simulink model "DIPC4M"  (R2015a)
settings: Solver=ode3  SolverMode=SingleTasking  StartTime=0.0  StopTime=3  FixedStep=1e-3  RelTol=1e-7
values from neighbouring files (symbols this model uses):
  alpha = 1.5    [CaViInit.m]    (also in CaccavaleVillani.m = 2)
  d1 = 1000    [CaViInit.m]    (also in CaccavaleVillani.m = 100)
  delta1 = 80    [CaViInit.m]    (also in CaccavaleVillani.m = 100)
  deltao = 10    [CaViInit.m]    (also in CaccavaleVillani.m = 2000)
  Do = 1500    [CaViInit.m]    (also in CaccavaleVillani.m = 2000)
  g = [0;0;-9.81]    [CaViInit.m]    (also in CaccavaleVillani.m)
  j0 = 0.2    [CaViInit.m]    (also in CaccavaleVillani.m = 1)
  j1 = 2    [CaViInit.m]    (also in CaccavaleVillani.m = 1)
  j1d = 1.00*j1    (= 2)    [CaViInit.m]    (also in CaccavaleVillani.m = 1)
  j2 = 2    [CaViInit.m]    (also in CaccavaleVillani.m = 1)
  j2d = 1.00*j2    (= 2)    [CaViInit.m]    (also in CaccavaleVillani.m = 1)
  j3 = 2    [CaViInit.m]    (also in CaccavaleVillani.m = 1)
  j3d = 1.00*j3    (= 2)    [CaViInit.m]    (also in CaccavaleVillani.m = 1)
  j4 = 2    [CaViInit.m]    (also in CaccavaleVillani.m = 1)
  j4d = 1.00*j4    (= 2)    [CaViInit.m]    (also in CaccavaleVillani.m = 1)
  k1 = 400    [CaViInit.m]    (also in CaccavaleVillani.m = 10000)
  K_o = 700    [CaViInit.m]    (also in CaccavaleVillani.m = 10000)
  kappa1 = 2    [CaViInit.m]    (also in CaccavaleVillani.m = 250)
  kappa_o = 5    [CaViInit.m]    (also in CaccavaleVillani.m = 10000)
  kpr = 150    [CaViInit.m]    (also in CaccavaleVillani.m = 10000)
  kpt = 50    [CaViInit.m]    (also in CaccavaleVillani.m = 50000)
  kv = 300    [CaccavaleVillani.m]
  m0 = 1.4    [CaViInit.m]    (also in CaccavaleVillani.m = 10)
  m1 = 2    [CaViInit.m]    (also in CaccavaleVillani.m = 10)
  m1d = 1.00*m1    (= 2)    [CaViInit.m]    (also in CaccavaleVillani.m = 10)
  m2 = 2    [CaViInit.m]    (also in CaccavaleVillani.m = 10)
  m2d = 1.00*m2    (= 2)    [CaViInit.m]    (also in CaccavaleVillani.m = 10)
  m3 = 2    [CaViInit.m]    (also in CaccavaleVillani.m = 10)
  m3d = 1.00*m3    (= 2)    [CaViInit.m]    (also in CaccavaleVillani.m = 10)
  m4 = 2    [CaViInit.m]    (also in CaccavaleVillani.m = 10)
  m4d = 1.00*m4    (= 2)    [CaViInit.m]    (also in CaccavaleVillani.m = 10)
  r = 0.4*[1; 0; 0 ... (first row only)    [CaViInit.m]    (also in CaccavaleVillani.m = [1; 0; 0)
libraries: aerolibutil x24, dspinverses x3, aerolibtransform2 x2, simulink x2
(part 1 of 2)
settings Model: CovSFcnEnable=off  Creator=Martin  LastModifiedBy=mangerer
settings SolverCC: ZeroCrossAlgorithm=Adaptive  AlgebraicLoopSolver=LineSearch
settings DataIOCC: LimitDataPoints=off
settings OptimizationCC: BlockReduction=off  BooleanDataType=off
settings DebuggingCC: SaveWithParameterizedLinksMsg=none  UnderspecifiedInitializationDetection=Classic  MergeDetectMultiDrivingBlocksExec=none  SignalResolutionControl=TryResolveAllWithWarning
settings HardwareCC: TargetUnknown=on

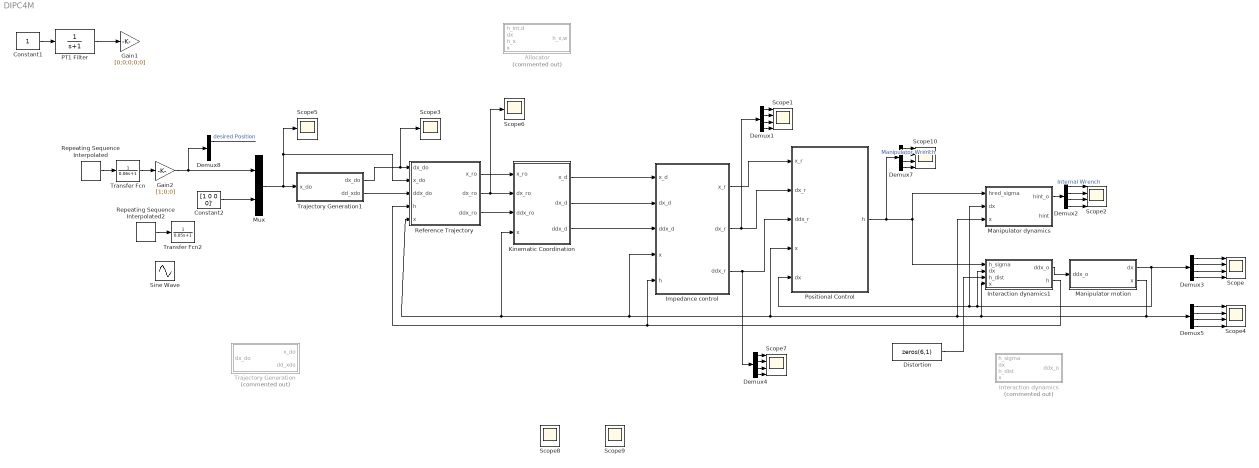
== system DIPC4M ==
  Allocator : Subsystem  Commented=on
  Constant1 : Constant
  Constant2 : Constant  Value=[1 0 0 0]'
  Demux{1..5,7} (6 alike) : Demux
  Demux8 : Demux  Outputs=3
  Distortion : Constant  Value=zeros(6,1)
  Gain1 : Gain  Gain=[0;0;0;0;0]
  Gain2 : Gain  Gain=[1;0;0]
  Impedance control : Subsystem
  Interaction dynamics : Subsystem  Commented=on
  Interaction dynamics1 : Subsystem
  Kinematic Coordination : Subsystem
  Manipulator dynamics : Subsystem
  Manipulator motion : Subsystem
  Mux : Mux  Inputs=2
  PT1 Filter : TransferFcn  Denominator=[1 1]
  Positional Control : Subsystem
  Reference Trajectory : Subsystem
  Repeating Sequence Interpolated : simulink/Sources/Repeating Sequence Interpolated  OutValues=[0 0 2 2 4 4 -2 -2 0 0].'  TimeValues=[0 0.1 0.14 0.9 0.96 1.8 1.95 2.4 2.6 3].'  LookUpMeth=Interpolation-Use End Values  tsamp=0.001  OutMin=[]  OutMax=[]  OutDataTypeStr=double  OutputDataTypeScalingMode=double  OutDataType=fixdt(0,8)  OutScaling=2^-10
  Repeating Sequence Interpolated2 : simulink/Sources/Repeating Sequence Interpolated  OutValues=[0 0 1 1 0 0].'  TimeValues=[0 0.1 1.5 2 2.5 3].'  LookUpMeth=Interpolation-Use End Values  tsamp=0.001  OutMin=[]  OutMax=[]  OutDataTypeStr=double  OutputDataTypeScalingMode=double  OutDataType=fixdt(0,8)  OutScaling=2^-10
  Scope{,1..2,4,7..10} (8 alike) : Scope  NumInputPorts=4
      Scope settings: ShowLegends=on  YMin=-1.5~-1.5~-1.5~-1.5  YMax=1.25~1.5~1.5~1.25
      Scope1 settings: ShowLegends=on  YMin=-2.5~-2.5~-3~-3  YMax=3~3~2.5~2.5
      Scope10 settings: ShowLegends=on  YMin=-30~-40~-40~-30  YMax=40~30~30~40  SaveName=ScopeData18
      Scope2 settings: ShowLegends=on  YMin=-1e-12~-1.5e-12~-7e-12~-3e-12  YMax=8e-12~3.5e-12~4e-12~4e-12  SaveName=ScopeData2
      Scope4 settings: ShowLegends=on  YMin=-1~-1~-0.5~-2  YMax=6~5~3.5~5  SaveName=ScopeData10
      Scope7 settings: ShowLegends=on  YMin=-3.5~-3.5~-3.5~-3.25  YMax=2~3~3~0.25  SaveName=ScopeData26
      Scope8 settings: Floating=on  ShowLegends=on  TimeRange=3  YMin=-3~-40~-10000~-0.005  YMax=5~30~10000~0.005  SaveName=ScopeData40
      Scope9 settings: Floating=on  ShowLegends=on  TimeRange=3  YMin=-0.2~-0.2~-30~-0.2  YMax=1.6~1.2~30~0.2  SaveName=ScopeData39
  Scope3 : Scope
      settings: SaveName=ScopeData8
  Scope5 : Scope
      settings: SaveName=ScopeData11
  Scope6 : Scope
      settings: YMin=-1  YMax=1  SaveName=ScopeData12
  Sine Wave : Sin  Frequency=1*pi  SampleTime=0
  Trajectory Generation : Subsystem  Commented=on
  Trajectory Generation1 : Subsystem
  Transfer Fcn : TransferFcn  Denominator=[0.06 1]
  Transfer Fcn2 : TransferFcn  Denominator=[0.05 1]
  wires:
  Manipulator dynamics/1(hint_o) -> Demux2/1
  Demux2/1 -> Scope2/1  "Internal Wrench"
  Demux2/2 -> Scope2/2
  Demux2/4 -> Scope2/4
  Demux3/1 -> Scope/1
  Demux3/2 -> Scope/2
  Demux3/3 -> Scope/3
  Demux3/4 -> Scope/4
  Demux5/1 -> Scope4/1
  Demux5/2 -> Scope4/2
  Demux5/3 -> Scope4/3
  Demux5/4 -> Scope4/4
  Demux7/1 -> Scope10/1  "Manipulator Wrench"
  Demux7/2 -> Scope10/2
  Demux7/3 -> Scope10/3
  Demux7/4 -> Scope10/4
  PT1 Filter/1 -> Gain1/1
  Manipulator motion/1(dx) -> Demux3/1, Positional Control/5(dx), Manipulator dynamics/2(dx), Interaction dynamics1/2(dx)
  Kinematic Coordination/1(x_d) -> Impedance control/1(x_d)
  Kinematic Coordination/3(ddx_d) -> Impedance control/3(ddx_d)
  Manipulator motion/2(x) -> Demux5/1, Interaction dynamics1/4(x), Manipulator dynamics/3(x), Positional Control/4(x), Kinematic Coordination/4(x), Reference Trajectory/5(x), Impedance control/4(x)
  Constant1/1 -> PT1 Filter/1
  Demux1/1 -> Scope1/1
  Demux1/2 -> Scope1/2
  Demux1/3 -> Scope1/3
  Demux1/4 -> Scope1/4
  Kinematic Coordination/2(dx_d) -> Impedance control/2(dx_d)
  Demux2/3 -> Scope2/3
  Interaction dynamics1/1(ddx_o) -> Manipulator motion/1(ddx_o)
  Distortion/1 -> Interaction dynamics1/3(h_dist)
  Reference Trajectory/1(x_ro) -> Kinematic Coordination/1(x_ro)
  Reference Trajectory/2(dx_ro) -> Scope6/1, Kinematic Coordination/2(dx_ro)
  Reference Trajectory/3(ddx_ro) -> Kinematic Coordination/3(ddx_ro)
  Impedance control/1(x_r) -> Positional Control/1(x_r)
  Impedance control/2(dx_r) -> Demux1/1, Positional Control/2(dx_r)
  Impedance control/3(ddx_r) -> Demux4/1, Positional Control/3(ddx_r)
  Positional Control/1(h) -> Demux7/1, Interaction dynamics1/1(h_sigma), Manipulator dynamics/1(hred_sigma)
  Demux4/1 -> Scope7/1
  Demux4/2 -> Scope7/2
  Demux4/3 -> Scope7/3
  Demux4/4 -> Scope7/4
  Repeating Sequence Interpolated2/1 -> Transfer Fcn2/1
  Mux/1 -> Scope5/1, Reference Trajectory/2(x_do), Trajectory Generation1/1(x_do)
  Trajectory Generation1/1(dx_do) -> Scope3/1, Reference Trajectory/1(dx_do)
  Trajectory Generation1/2(dd_xdo) -> Reference Trajectory/3(ddx_do)
  Gain2/1 -> Mux/1, Demux8/1
  Repeating Sequence Interpolated/1 -> Transfer Fcn/1
  Transfer Fcn/1 -> Gain2/1
  Demux8/1 -> ?  "desired Position"
  Constant2/1 -> Mux/2
  Interaction dynamics1/2(h) -> Reference Trajectory/4(h), Impedance control/5(h)

== system DIPC4M/Allocator ==
  h_int,d : Inport
  dx : Inport  Port=2
  h_x : Inport  Port=3
  x : Inport  Port=4
  Add : Sum  Inputs=-+
  Add1 : Sum
  Divide : Product  Inputs=*/*  Multiplication=Matrix(*)
  Divide1 : Product  Inputs=*/*  Multiplication=Matrix(*)
  Divide2 : Product  Inputs=*/*  Multiplication=Matrix(*)
  Inertia : Constant  Value=blkdiag(m1d*eye(3), j1d*eye(3), m2d*eye(3), j2d*eye(3), m3d*eye(3), j3d*eye(3), m4d*eye(3), j4d*eye(3))
  MATLAB Function : MATLAB Function  TreatAsAtomicUnit=on
  MATLAB Function1 : MATLAB Function  TreatAsAtomicUnit=on
  Math Function : Math  Operator=transpose  SaturateOnIntegerOverflow=on
  h_x,w : Outport
  wires:
  dx/1 -> MATLAB Function1/1(dx)
  Divide/1 -> h_x,w/1
  Math Function/1 -> Divide1/3, Divide/1
  MATLAB Function/1(Ared) -> Math Function/1, Divide2/1, Divide1/1
  Divide1/1 -> Divide/2
  Inertia/1 -> Divide1/2, Divide2/2
  MATLAB Function1/1(bred) -> Add/2
  Add/1 -> Divide/3
  Divide2/1 -> Add/1
  Add1/1 -> Divide2/3
  h_int,d/1 -> Add1/1
  h_x/1 -> Add1/2
  x/1 -> MATLAB Function1/2(x), MATLAB Function/1(x)

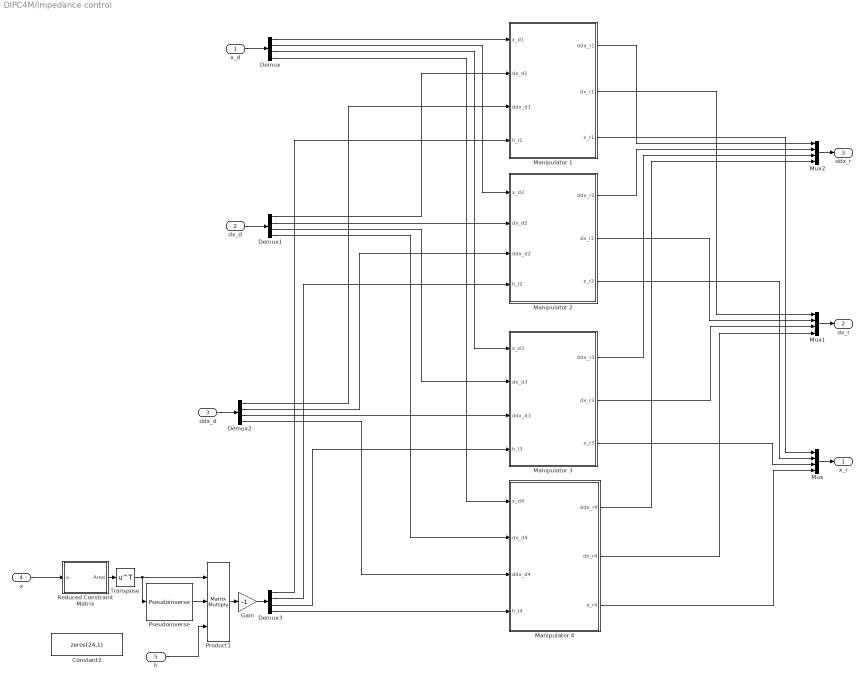
== system DIPC4M/Impedance control ==
  x_d : Inport
  dx_d : Inport  Port=2
  ddx_d : Inport  Port=3
  x : Inport  Port=4
  h : Inport  Port=5
  Constant2 : Constant  Value=zeros(24,1)
  Demux{,1..3} (4 alike) : Demux
  Gain : Gain  Gain=-1
  Manipulator 1 : Subsystem
  Manipulator 2 : Subsystem
  Manipulator 3 : Subsystem
  Manipulator 4 : Subsystem
  Mux : Mux
  Mux1 : Mux
  Mux2 : Mux
  Product1 : Product  Inputs=***  Multiplication=Matrix(*)
  Pseudoinverse : dspinverses/Pseudoinverse  wanterr=off
  Reduced Constraint Matrix : MATLAB Function  TreatAsAtomicUnit=on
  Transpose : Math  Operator=transpose  SaturateOnIntegerOverflow=on
  x_r : Outport
  dx_r : Outport  Port=2
  ddx_r : Outport  Port=3
  wires:
  ddx_d/1 -> Demux2/1
  dx_d/1 -> Demux1/1
  x_d/1 -> Demux/1
  Mux/1 -> x_r/1
  x/1 -> Reduced Constraint Matrix/1(x)
  Demux/1 -> Manipulator 1/1(x_d1)
  Demux/2 -> Manipulator 2/1(x_d2)
  Demux/3 -> Manipulator 3/1(x_d3)
  Demux1/1 -> Manipulator 1/2(dx_d1)
  Demux1/2 -> Manipulator 2/2(dx_d2)
  Demux1/3 -> Manipulator 3/2(dx_d3)
  Demux1/4 -> Manipulator 4/2(dx_d4)
  Demux/4 -> Manipulator 4/1(x_d4)
  Demux2/1 -> Manipulator 1/3(ddx_d1)
  Demux2/2 -> Manipulator 2/3(ddx_d2)
  Demux2/3 -> Manipulator 3/3(ddx_d3)
  Demux2/4 -> Manipulator 4/3(ddx_d4)
  Demux3/1 -> Manipulator 1/4(h_I1)
  Demux3/2 -> Manipulator 2/4(h_I2)
  Demux3/3 -> Manipulator 3/4(h_I3)
  Demux3/4 -> Manipulator 4/4(h_I4)
  Mux1/1 -> dx_r/1
  Mux2/1 -> ddx_r/1
  Manipulator 1/1(ddx_r1) -> Mux2/1
  Manipulator 2/1(ddx_r2) -> Mux2/2
  Manipulator 3/1(ddx_r3) -> Mux2/3
  Manipulator 4/1(ddx_r4) -> Mux2/4
  Manipulator 1/2(dx_r1) -> Mux1/1
  Manipulator 2/2(dx_r2) -> Mux1/2
  Manipulator 3/2(dx_r3) -> Mux1/3
  Manipulator 4/2(dx_r4) -> Mux1/4
  Manipulator 4/3(x_r4) -> Mux/4
  Manipulator 3/3(x_r3) -> Mux/3
  Manipulator 2/3(x_r2) -> Mux/2
  Manipulator 1/3(x_r1) -> Mux/1
  Pseudoinverse/1 -> Product1/2
  Reduced Constraint Matrix/1(Ared) -> Transpose/1
  Transpose/1 -> Product1/1, Pseudoinverse/1
  Product1/1 -> Gain/1
  Gain/1 -> Demux3/1
  h/1 -> Product1/3

== system DIPC4M/Interaction dynamics ==
  h_sigma : Inport
  dx : Inport  Port=2
  h_dist : Inport  Port=3
  x : Inport  Port=4
  Apparent Inertia : MATLAB Function  TreatAsAtomicUnit=on
  Centripetal Force : MATLAB Function  TreatAsAtomicUnit=on
  Coriolis Force : MATLAB Function  TreatAsAtomicUnit=on
  G h_sigma : Product  Multiplication=Matrix(*)
  GMb : Product  Inputs=***  Multiplication=Matrix(*)
  Grasp Matrix : MATLAB Function  TreatAsAtomicUnit=on
  Gravitation : Constant  Value=[-m0*g;zeros(3,1)]
  Inertia : Constant  Value=blkdiag(m1*eye(3), j1*eye(3), m2*eye(3), j2*eye(3), m3*eye(3), j3*eye(3), m4*eye(3), j4*eye(3))
  M_app^-1 h_o : Product  Inputs=/*  Multiplication=Matrix(*)
  "h_dist - h_g - j0 S(omega0) omega0 " : Sum  Inputs=+--
  h_o : Sum  Inputs=++-
  ddx_o : Outport
  wires:
  Grasp Matrix/1(G) -> G h_sigma/1, GMb/1, Apparent Inertia/1(G)
  Inertia/1 -> GMb/2, Apparent Inertia/2(M)
  Apparent Inertia/1(Mapp) -> M_app^-1 h_o/1
  h_o/1 -> M_app^-1 h_o/2
  G h_sigma/1 -> h_o/2
  h_sigma/1 -> G h_sigma/2
  "h_dist - h_g - j0 S(omega0) omega0 "/1 -> h_o/1
  h_dist/1 -> "h_dist - h_g - j0 S(omega0) omega0 "/1
  Gravitation/1 -> "h_dist - h_g - j0 S(omega0) omega0 "/2
  dx/1 -> Centripetal Force/1(dx), Coriolis Force/1(dx)
  Coriolis Force/1(hcoriolis) -> "h_dist - h_g - j0 S(omega0) omega0 "/3
  GMb/1 -> h_o/3
  Centripetal Force/1(b) -> GMb/3
  M_app^-1 h_o/1 -> ddx_o/1
  x/1 -> Centripetal Force/2(x), Grasp Matrix/1(x)

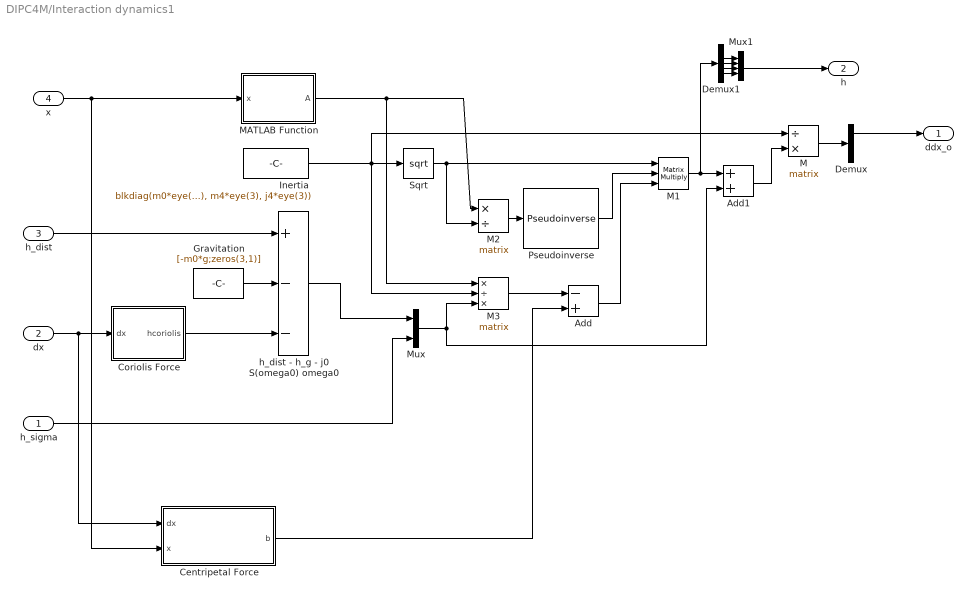
== system DIPC4M/Interaction dynamics1 ==
  h_sigma : Inport
  dx : Inport  Port=2
  h_dist : Inport  Port=3
  x : Inport  Port=4
  Add : Sum  Inputs=-+
  Add1 : Sum
  Centripetal Force : MATLAB Function  TreatAsAtomicUnit=on
  Coriolis Force : MATLAB Function  TreatAsAtomicUnit=on
  Demux : Demux  Outputs=5
  Demux1 : Demux  Outputs=5
  Gravitation : Constant  Value=[-m0*g;zeros(3,1)]
  Inertia : Constant  Value=blkdiag(m0*eye(3),j0*eye(3),m1*eye(3), j1*eye(3), m2*eye(3), j2*eye(3), m3*eye(3), j3*eye(3), m4*eye(3), j4*eye(3))
  M : Product  Inputs=/*  Multiplication=Matrix(*)
  M1 : Product  Inputs=***  Multiplication=Matrix(*)
  M2 : Product  Inputs=*/  Multiplication=Matrix(*)
  M3 : Product  Inputs=*/*  Multiplication=Matrix(*)
  MATLAB Function : MATLAB Function  TreatAsAtomicUnit=on
  Mux : Mux  Inputs=2
  Mux1 : Mux
  Pseudoinverse : dspinverses/Pseudoinverse  wanterr=off
  Sqrt : Sqrt  SaturateOnIntegerOverflow=on
  "h_dist - h_g - j0 S(omega0) omega0 " : Sum  Inputs=+--
  ddx_o : Outport
  h : Outport  Port=2
  wires:
  h_dist/1 -> "h_dist - h_g - j0 S(omega0) omega0 "/1
  Gravitation/1 -> "h_dist - h_g - j0 S(omega0) omega0 "/2
  dx/1 -> Centripetal Force/1(dx), Coriolis Force/1(dx)
  Coriolis Force/1(hcoriolis) -> "h_dist - h_g - j0 S(omega0) omega0 "/3
  x/1 -> MATLAB Function/1(x), Centripetal Force/2(x)
  Inertia/1 -> M/1, M3/2, Sqrt/1
  Sqrt/1 -> M2/2, M1/1
  MATLAB Function/1(A) -> M3/1, M2/1
  M2/1 -> Pseudoinverse/1
  Pseudoinverse/1 -> M1/2
  Add/1 -> M1/3
  Centripetal Force/1(b) -> Add/2
  M3/1 -> Add/1
  Mux/1 -> Add1/2, M3/3
  "h_dist - h_g - j0 S(omega0) omega0 "/1 -> Mux/1
  h_sigma/1 -> Mux/2
  M/1 -> Demux/1
  Demux/1 -> ddx_o/1
  M1/1 -> Demux1/1, Add1/1
  Add1/1 -> M/2
  Demux1/2 -> Mux1/1
  Demux1/3 -> Mux1/2
  Demux1/4 -> Mux1/3
  Demux1/5 -> Mux1/4
  Mux1/1 -> h/1

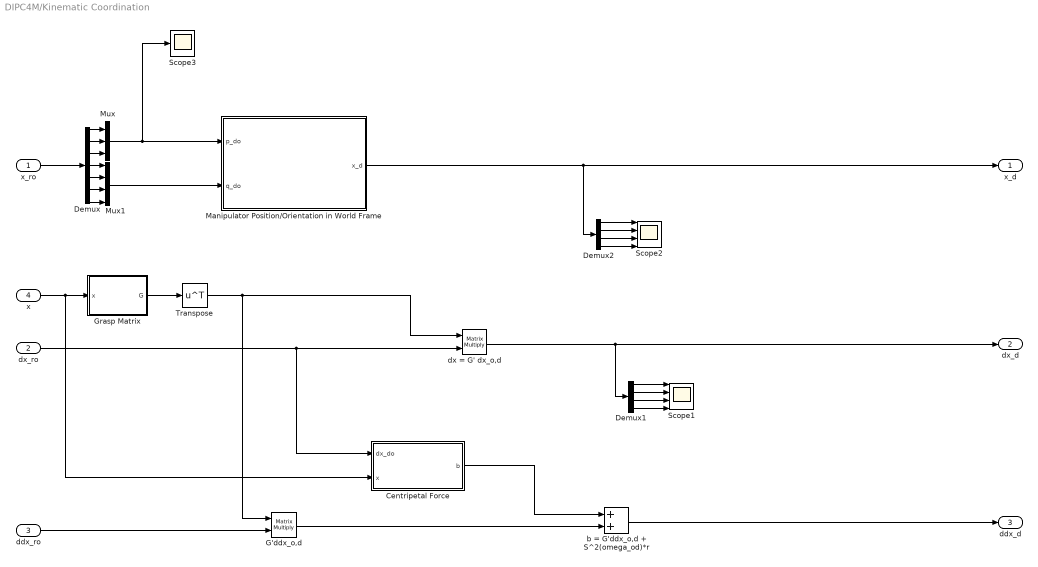
== system DIPC4M/Kinematic Coordination ==
  x_ro : Inport
  dx_ro : Inport  Port=2
  ddx_ro : Inport  Port=3
  x : Inport  Port=4
  Centripetal Force : MATLAB Function  TreatAsAtomicUnit=on
  Demux : Demux  Outputs=7
  Demux1 : Demux
  Demux2 : Demux
  G'ddx_o,d : Product  Multiplication=Matrix(*)
  Grasp Matrix : MATLAB Function  TreatAsAtomicUnit=on
  Manipulator Position/Orientation in World Frame : MATLAB Function  TreatAsAtomicUnit=on
  Mux : Mux  Inputs=3
  Mux1 : Mux
  Scope1 : Scope  NumInputPorts=4
      settings: ShowLegends=on  YMin=-1.5~-1.5~-1.5~-1.5  YMax=6~5.5~6~5.5  SaveName=ScopeData3
  Scope2 : Scope  NumInputPorts=4
      settings: ShowLegends=on  YMin=-1.5~-1.5~-1.5~-1.5  YMax=6~5.5~6~5.5  SaveName=ScopeData4
  Scope3 : Scope
      settings: ShowLegends=on  TimeRange=5  YMin=-0.25  YMax=0.175  SaveName=ScopeData30
  Transpose : Math  Operator=transpose  SaturateOnIntegerOverflow=on
  b = G'ddx_o,d + S^2(omega_od)*r : Sum
  dx = G' dx_o,d : Product  Multiplication=Matrix(*)
  x_d : Outport
  dx_d : Outport  Port=2
  ddx_d : Outport  Port=3
  wires:
  Grasp Matrix/1(G) -> Transpose/1
  Transpose/1 -> G'ddx_o,d/1, dx = G' dx_o,d/1
  dx = G' dx_o,d/1 -> Demux1/1, dx_d/1
  x_ro/1 -> Demux/1
  Demux/1 -> Mux/1
  Demux/2 -> Mux/2
  Demux/3 -> Mux/3
  Demux/5 -> Mux1/2
  Demux/6 -> Mux1/3
  Demux/7 -> Mux1/4
  Demux/4 -> Mux1/1
  Mux1/1 -> Manipulator Position/Orientation in World Frame/2(q_do)
  Mux/1 -> Scope3/1, Manipulator Position/Orientation in World Frame/1(p_do)
  Centripetal Force/1(b) -> b = G'ddx_o,d + S^2(omega_od)*r/1
  ddx_ro/1 -> G'ddx_o,d/2
  G'ddx_o,d/1 -> b = G'ddx_o,d + S^2(omega_od)*r/2
  b = G'ddx_o,d + S^2(omega_od)*r/1 -> ddx_d/1
  dx_ro/1 -> Centripetal Force/1(dx_do), dx = G' dx_o,d/2
  Demux1/1 -> Scope1/1
  Demux1/2 -> Scope1/2
  Demux1/3 -> Scope1/3
  Demux1/4 -> Scope1/4
  Manipulator Position/Orientation in World Frame/1(x_d) -> Demux2/1, x_d/1
  Demux2/1 -> Scope2/1
  Demux2/2 -> Scope2/2
  Demux2/3 -> Scope2/3
  Demux2/4 -> Scope2/4
  x/1 -> Centripetal Force/2(x), Grasp Matrix/1(x)

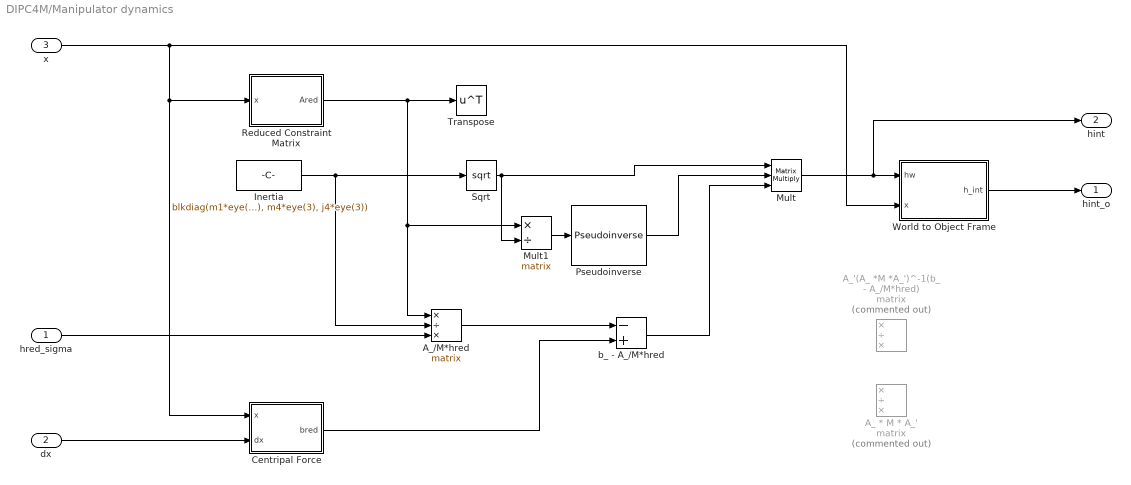
== system DIPC4M/Manipulator dynamics ==
  hred_sigma : Inport
  dx : Inport  Port=2
  x : Inport  Port=3
  A_ * M * A_' : Product  Commented=on  Inputs=*/*  Multiplication=Matrix(*)
  A_'(A_ *M *A_')^-1(b_ - A_/M*hred) : Product  Commented=on  Inputs=*/*  Multiplication=Matrix(*)
  A_/M*hred : Product  Inputs=*/*  Multiplication=Matrix(*)
  Centripal Force : MATLAB Function  TreatAsAtomicUnit=on
  Inertia : Constant  Value=blkdiag(m1*eye(3), j1*eye(3), m2*eye(3), j2*eye(3), m3*eye(3), j3*eye(3), m4*eye(3), j4*eye(3))
  Mult : Product  Inputs=***  Multiplication=Matrix(*)
  Mult1 : Product  Inputs=*/  Multiplication=Matrix(*)
  Pseudoinverse : dspinverses/Pseudoinverse  wanterr=off
  Reduced Constraint Matrix : MATLAB Function  TreatAsAtomicUnit=on
  Sqrt : Sqrt  SaturateOnIntegerOverflow=on
  Transpose : Math  Operator=transpose  SaturateOnIntegerOverflow=on
  World to Object Frame : MATLAB Function  TreatAsAtomicUnit=on
  b_ - A_/M*hred : Sum  Inputs=-+
  hint_o : Outport
  hint : Outport  Port=2
  wires:
  Reduced Constraint Matrix/1(Ared) -> Transpose/1, A_/M*hred/1, Mult1/1
  Inertia/1 -> Sqrt/1, A_/M*hred/2
  dx/1 -> Centripal Force/2(dx)
  A_/M*hred/1 -> b_ - A_/M*hred/1
  hred_sigma/1 -> A_/M*hred/3
  World to Object Frame/1(h_int) -> hint_o/1
  x/1 -> Centripal Force/1(x), Reduced Constraint Matrix/1(x), World to Object Frame/2(x)
  Centripal Force/1(bred) -> b_ - A_/M*hred/2
  Mult/1 -> hint/1, World to Object Frame/1(hw)
  b_ - A_/M*hred/1 -> Mult/3
  Sqrt/1 -> Mult1/2, Mult/1
  Mult1/1 -> Pseudoinverse/1
  Pseudoinverse/1 -> Mult/2

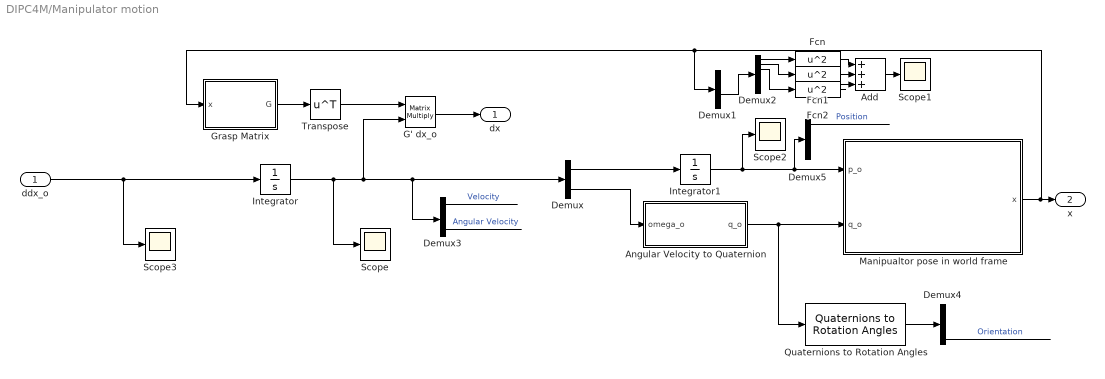
== system DIPC4M/Manipulator motion ==
  ddx_o : Inport
  Add : Sum  Inputs=+++
  Angular Velocity to Quaternion : Subsystem
  Demux : Demux  Outputs=2
  Demux1 : Demux
  Demux2 : Demux  Outputs=7
  Demux3 : Demux  Outputs=6
  Demux4 : Demux  Outputs=3
  Demux5 : Demux  Outputs=3
  Fcn : Fcn  Expr=u^2
  Fcn1 : Fcn  Expr=u^2
  Fcn2 : Fcn  Expr=u^2
  G' dx_o : Product  Multiplication=Matrix(*)
  Grasp Matrix : MATLAB Function  TreatAsAtomicUnit=on
  Integrator : Integrator  InitialCondition=zeros(6,1)
  Integrator1 : Integrator  InitialCondition=[0 0 0]'
  Manipualtor pose in world frame : MATLAB Function  TreatAsAtomicUnit=on
  Quaternions to Rotation Angles : aerolibtransform2/Quaternions to Rotation Angles  rotationOrder=XYZ
  Scope{,1..3} (4 alike) : Scope
      Scope settings: YMin=-1.1  YMax=1.1  SaveName=ScopeData14
      Scope1 settings: YMin=0  YMax=40  SaveName=ScopeData15
      Scope2 settings: YMin=-1  YMax=1  SaveName=ScopeData6
      Scope3 settings: SaveName=ScopeData7
  Transpose : Math  Operator=transpose  SaturateOnIntegerOverflow=on
  dx : Outport
  x : Outport  Port=2
  wires:
  ddx_o/1 -> Scope3/1, Integrator/1
  Integrator/1 -> Scope/1, G' dx_o/2, Demux3/1, Demux/1
  Grasp Matrix/1(G) -> Transpose/1
  Transpose/1 -> G' dx_o/1
  G' dx_o/1 -> dx/1
  Demux/2 -> Angular Velocity to Quaternion/1(omega_o)
  Demux/1 -> Integrator1/1
  Integrator1/1 -> Scope2/1, Demux5/1, Manipualtor pose in world frame/1(p_o)
  Manipualtor pose in world frame/1(x) -> Demux1/1, Grasp Matrix/1(x), x/1
  Angular Velocity to Quaternion/1(q_o) -> Quaternions to Rotation Angles/1, Manipualtor pose in world frame/2(q_o)
  Add/1 -> Scope1/1
  Fcn/1 -> Add/1
  Fcn1/1 -> Add/2
  Fcn2/1 -> Add/3
  Demux2/1 -> Fcn/1
  Demux2/2 -> Fcn1/1
  Demux2/3 -> Fcn2/1
  Demux1/3 -> Demux2/1
  Demux3/1 -> ?  "Velocity"
  Quaternions to Rotation Angles/1 -> Demux4/1
  Demux4/3 -> ?  "Orientation"
  Demux3/6 -> ?  "Angular Velocity"
  Demux5/1 -> ?  "Position"

== system DIPC4M/Positional Control ==
  x_r : Inport
  dx_r : Inport  Port=2
  ddx_r : Inport  Port=3
  x : Inport  Port=4
  dx : Inport  Port=5
  Add : Sum  Inputs=+++
  Add1 : Sum  Inputs=+-
  Manipulator Inertia : Constant  Value=blkdiag(m1*eye(3), j1*eye(3), m2*eye(3), j2*eye(3), m3*eye(3), j3*eye(3), m4*eye(3), j4*eye(3))
  Manipulator kv : Constant  Value=kv*eye(24)
  Product : Product  Multiplication=Matrix(*)
  Product1 : Product  Multiplication=Matrix(*)
  Subsystem : Subsystem
  h : Outport
  wires:
  Product/1 -> h/1
  Manipulator Inertia/1 -> Product/1
  Add/1 -> Product/2
  ddx_r/1 -> Add/3
  dx_r/1 -> Add1/1
  dx/1 -> Add1/2
  x/1 -> Subsystem/2(x)
  x_r/1 -> Subsystem/1(x_r)
  Subsystem/1(hk) -> Add/1
  Add1/1 -> Product1/2
  Manipulator kv/1 -> Product1/1
  Product1/1 -> Add/2

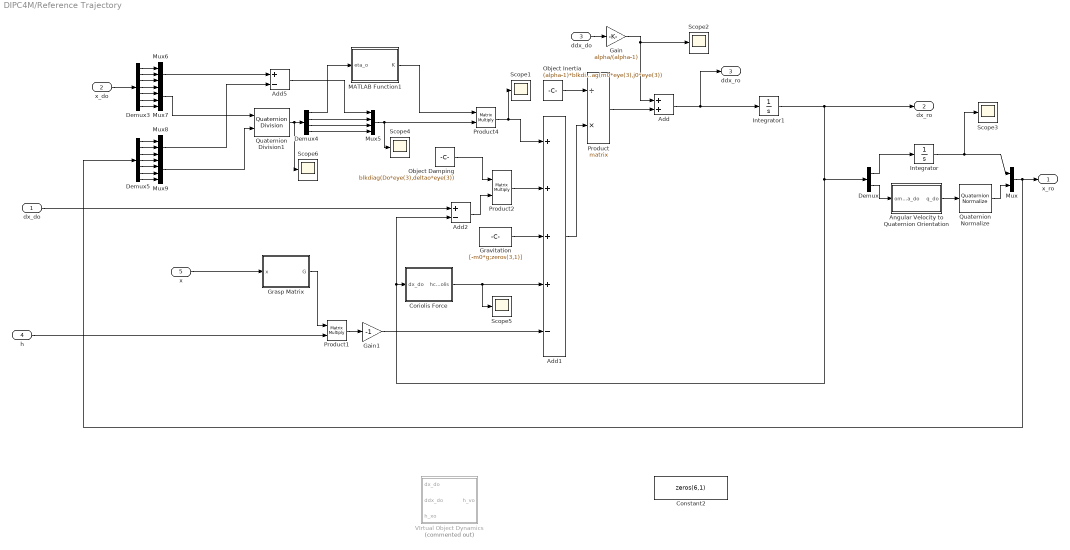
== system DIPC4M/Reference Trajectory ==
  dx_do : Inport
  x_do : Inport  Port=2
  ddx_do : Inport  Port=3
  h : Inport  Port=4
  x : Inport  Port=5
  Add : Sum
  Add1 : Sum  Inputs=++++-
  Add2 : Sum  Inputs=+-
  Add5 : Sum  Inputs=+-
  Angular Velocity to Quaternion Orientation : Subsystem
  Constant2 : Constant  Value=zeros(6,1)
  Coriolis Force : MATLAB Function  TreatAsAtomicUnit=on
  Demux : Demux  Outputs=2
  Demux3 : Demux  Outputs=7
  Demux4 : Demux
  Demux5 : Demux  Outputs=7
  Gain : Gain  Gain=alpha/(alpha-1)
  Gain1 : Gain  Gain=-1
  Grasp Matrix : MATLAB Function  TreatAsAtomicUnit=on
  Gravitation : Constant  Value=[-m0*g;zeros(3,1)]
  Integrator : Integrator  InitialCondition=zeros(3,1)
  Integrator1 : Integrator  InitialCondition=zeros(6,1)
  MATLAB Function1 : MATLAB Function  TreatAsAtomicUnit=on
  Mux : Mux  Inputs=2
  Mux5 : Mux
  Mux6 : Mux  Inputs=3
  Mux7 : Mux
  Mux8 : Mux  Inputs=3
  Mux9 : Mux
  Object Damping : Constant  Value=blkdiag(Do*eye(3),deltao*eye(3))
  Object Inertia : Constant  Value=(alpha-1)*blkdiag(m0*eye(3),j0*eye(3))
  Product : Product  Inputs=/*  Multiplication=Matrix(*)
  Product1 : Product  Multiplication=Matrix(*)
  Product2 : Product  Multiplication=Matrix(*)
  Product4 : Product  Multiplication=Matrix(*)
  Quaternion Division1 : aerolibutil/Quaternion Division
  Quaternion Normalize : aerolibutil/Quaternion Normalize
  Scope{1..6} (6 alike) : Scope
      Scope1 settings: YMin=-325  YMax=100  SaveName=ScopeData23
      Scope2 settings: SaveName=ScopeData25
      Scope3 settings: ShowLegends=on  TimeRange=5  YMin=-0.15  YMax=0.01  SaveName=ScopeData31
      Scope4 settings: YMin=-0.4  YMax=0.25  SaveName=ScopeData27
      Scope5 settings: ShowLegends=on  TimeRange=5  YMin=-15  YMax=12.5  SaveName=ScopeData32
      Scope6 settings: YMin=-0.05  YMax=1  SaveName=ScopeData28
  VIrtual Object Dynamics : Subsystem  Commented=on
  x_ro : Outport
  dx_ro : Outport  Port=2
  ddx_ro : Outport  Port=3
  wires:
  Object Inertia/1 -> Product/1
  Add/1 -> ddx_ro/1, Integrator1/1
  Add1/1 -> Product/2
  MATLAB Function1/1(K) -> Product4/1
  Demux4/1 -> MATLAB Function1/1(eta_o)
  Add5/1 -> Mux5/1
  Demux4/2 -> Mux5/2
  Demux4/3 -> Mux5/3
  Demux4/4 -> Mux5/4
  x_do/1 -> Demux3/1
  Demux3/2 -> Mux6/2
  Demux3/1 -> Mux6/1
  Demux3/3 -> Mux6/3
  Demux3/4 -> Mux7/1
  Demux3/5 -> Mux7/2
  Demux3/6 -> Mux7/3
  Demux3/7 -> Mux7/4
  Demux5/2 -> Mux8/2
  Demux5/1 -> Mux8/1
  Demux5/3 -> Mux8/3
  Demux5/4 -> Mux9/1
  Demux5/5 -> Mux9/2
  Demux5/6 -> Mux9/3
  Demux5/7 -> Mux9/4
  Quaternion Division1/1 -> Scope6/1, Demux4/1
  Mux5/1 -> Scope4/1, Product4/2
  Product4/1 -> Scope1/1, Add1/1
  Mux6/1 -> Add5/1
  Mux7/1 -> Quaternion Division1/1
  Mux8/1 -> Add5/2
  Demux/2 -> Angular Velocity to Quaternion Orientation/1(omega_do)
  Demux/1 -> Integrator/1
  Integrator/1 -> Scope3/1, Mux/1
  Mux/1 -> Demux5/1, x_ro/1
  Grasp Matrix/1(G) -> Product1/1
  ddx_do/1 -> Gain/1
  Gain/1 -> Scope2/1, Add/1
  Product/1 -> Add/2
  Product2/1 -> Add1/2
  Object Damping/1 -> Product2/1
  Add2/1 -> Product2/2
  dx_do/1 -> Add2/1
  Gravitation/1 -> Add1/3
  Coriolis Force/1(hcoriolis) -> Scope5/1, Add1/4
  Integrator1/1 -> Add2/2, Coriolis Force/1(dx_do), Demux/1, dx_ro/1
  x/1 -> Grasp Matrix/1(x)
  Angular Velocity to Quaternion Orientation/1(q_do) -> Quaternion Normalize/1
  Mux9/1 -> Quaternion Division1/2
  Quaternion Normalize/1 -> Mux/2
  Product1/1 -> Gain1/1
  Gain1/1 -> Add1/5
  h/1 -> Product1/2

== system DIPC4M/Trajectory Generation ==
  dx_do : Inport
  Angular Velocity to Quaternion Orientation : Subsystem
  Demux : Demux  Outputs=2
  Demux4 : Demux  Outputs=3
  Derivative : Derivative
  Integrator : Integrator  InitialCondition=zeros(3,1)
  Mux : Mux  Inputs=2
  Quaternion Normalize : aerolibutil/Quaternion Normalize
  Quaternions to Rotation Angles : aerolibtransform2/Quaternions to Rotation Angles  rotationOrder=XYZ
  Scope : Scope
      settings: SaveName=ScopeData16
  x_do : Outport
  dd_xdo : Outport  Port=2
  wires:
  dx_do/1 -> Derivative/1, Demux/1
  Demux/2 -> Angular Velocity to Quaternion Orientation/1(omega_do)
  Demux/1 -> Integrator/1
  Angular Velocity to Quaternion Orientation/1(q_do) -> Quaternion Normalize/1
  Integrator/1 -> Mux/1
  Mux/1 -> x_do/1
  Derivative/1 -> dd_xdo/1
  Quaternion Normalize/1 -> Quaternions to Rotation Angles/1, Scope/1, Mux/2
  Quaternions to Rotation Angles/1 -> Demux4/1
  Demux4/3 -> ?  "desired Orientation"

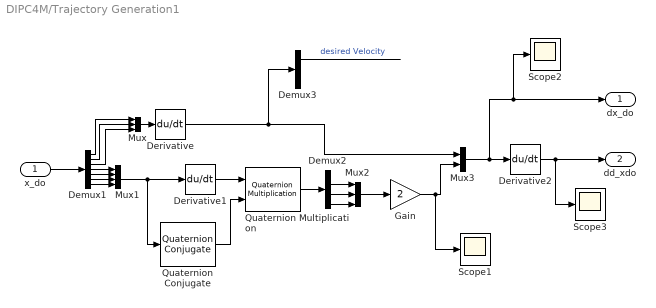
== system DIPC4M/Trajectory Generation1 ==
  x_do : Inport
  Demux1 : Demux  Outputs=7
  Demux2 : Demux
  Demux3 : Demux  Outputs=3
  Derivative : Derivative
  Derivative1 : Derivative
  Derivative2 : Derivative
  Gain : Gain  Gain=2
  Mux : Mux  Inputs=3
  Mux1 : Mux
  Mux2 : Mux  Inputs=3
  Mux3 : Mux  Inputs=2
  Quaternion Conjugate : aerolibutil/Quaternion Conjugate
  Quaternion Multiplication : aerolibutil/Quaternion Multiplication
  Scope1 : Scope
      settings: ShowLegends=on  YMin=0  YMax=2  SaveName=ScopeData10
  Scope2 : Scope
      settings: YMin=0  YMax=2  SaveName=ScopeData11
  Scope3 : Scope
      settings: YMin=-1.5e-09  YMax=1.5e-09  SaveName=ScopeData8
  dx_do : Outport
  dd_xdo : Outport  Port=2
  wires:
  x_do/1 -> Demux1/1
  Demux1/1 -> Mux/1
  Demux1/2 -> Mux/2
  Demux1/3 -> Mux/3
  Demux1/4 -> Mux1/1
  Demux1/5 -> Mux1/2
  Demux1/6 -> Mux1/3
  Demux1/7 -> Mux1/4
  Mux/1 -> Derivative/1
  Mux1/1 -> Quaternion Conjugate/1, Derivative1/1
  Derivative1/1 -> Quaternion Multiplication/1
  Quaternion Conjugate/1 -> Quaternion Multiplication/2
  Quaternion Multiplication/1 -> Demux2/1
  Demux2/4 -> Mux2/3
  Demux2/3 -> Mux2/2
  Demux2/2 -> Mux2/1
  Mux2/1 -> Gain/1
  Gain/1 -> Scope1/1, Mux3/2
  Derivative/1 -> Demux3/1, Mux3/1
  Mux3/1 -> Scope2/1, dx_do/1, Derivative2/1
  Derivative2/1 -> Scope3/1, dd_xdo/1
  Demux3/1 -> ?  "desired Velocity"

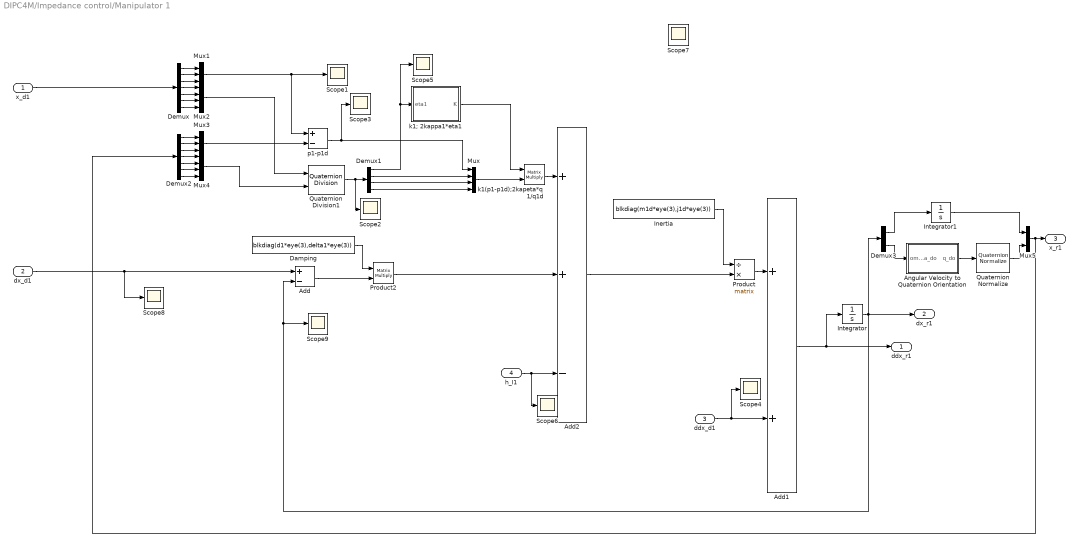
== system DIPC4M/Impedance control/Manipulator 1 ==
  x_d1 : Inport
  dx_d1 : Inport  Port=2
  ddx_d1 : Inport  Port=3
  h_I1 : Inport  Port=4
  Add : Sum  Inputs=+-
  Add1 : Sum
  Add2 : Sum  Inputs=++-
  Angular Velocity to Quaternion Orientation : Subsystem
  Damping : Constant  Value=blkdiag(d1*eye(3),delta1*eye(3))
  Demux : Demux  Outputs=7
  Demux1 : Demux
  Demux2 : Demux  Outputs=7
  Demux3 : Demux  Outputs=2
  Inertia : Constant  Value=blkdiag(m1d*eye(3),j1d*eye(3))
  Integrator : Integrator
  Integrator1 : Integrator  InitialCondition=r(1:3)
  Mux : Mux
  Mux1 : Mux  Inputs=3
  Mux2 : Mux
  Mux3 : Mux  Inputs=3
  Mux4 : Mux
  Mux5 : Mux  Inputs=2
  Product : Product  Inputs=/*  Multiplication=Matrix(*)
  Product2 : Product  Multiplication=Matrix(*)
  Quaternion Division1 : aerolibutil/Quaternion Division
  Quaternion Normalize : aerolibutil/Quaternion Normalize
  Scope{1..9} (9 alike) : Scope
      Scope1 settings: ShowLegends=on  TimeRange=5  YMin=2.77556e-17  YMax=1.05  SaveName=ScopeData29
      Scope2 settings: ShowLegends=on  TimeRange=5  YMin=-0.18  YMax=0.01  SaveName=ScopeData33
      Scope3 settings: ShowLegends=on  TimeRange=5  YMin=-0.18  YMax=0.01  SaveName=ScopeData21
      Scope4 settings: ShowLegends=on  TimeRange=5  YMin=-3.5  YMax=3  SaveName=ScopeData34
      Scope5 settings: ShowLegends=on  TimeRange=200  YMin=-50  YMax=125  SaveName=ScopeData24
      Scope6 settings: ShowLegends=on  TimeRange=5  YMin=-2.75e+09  YMax=1.5e+09  SaveName=ScopeData35
      Scope7 settings: ShowLegends=on  TimeRange=5  YMin=-0.18  YMax=0.01  SaveName=ScopeData36
      Scope8 settings: ShowLegends=on  TimeRange=5  YMin=-0.4  YMax=1.1  SaveName=ScopeData37
      Scope9 settings: ShowLegends=on  TimeRange=5  YMin=-1.1  YMax=1.1  SaveName=ScopeData38
  k1(p1-p1d);2kapeta*q1/q1d : Product  Multiplication=Matrix(*)
  k1; 2kappa1*eta1 : MATLAB Function  TreatAsAtomicUnit=on
  p1-p1d : Sum  Inputs=+-
  ddx_r1 : Outport
  dx_r1 : Outport  Port=2
  x_r1 : Outport  Port=3
  wires:
  Add/1 -> Product2/2
  Damping/1 -> Product2/1
  dx_d1/1 -> Scope8/1, Add/1
  k1; 2kappa1*eta1/1(K) -> k1(p1-p1d);2kapeta*q1/q1d/1
  Demux1/1 -> Scope5/1, k1; 2kappa1*eta1/1(eta1)
  p1-p1d/1 -> Scope3/1, Mux/1
  Demux1/2 -> Mux/2
  Demux1/3 -> Mux/3
  Demux1/4 -> Mux/4
  x_d1/1 -> Demux/1
  Demux/2 -> Mux1/2
  Demux/1 -> Mux1/1
  Demux/3 -> Mux1/3
  Demux/4 -> Mux2/1
  Demux/5 -> Mux2/2
  Demux/6 -> Mux2/3
  Demux/7 -> Mux2/4
  Demux2/2 -> Mux3/2
  Demux2/1 -> Mux3/1
  Demux2/3 -> Mux3/3
  Demux2/4 -> Mux4/1
  Demux2/5 -> Mux4/2
  Demux2/6 -> Mux4/3
  Demux2/7 -> Mux4/4
  Mux1/1 -> Scope1/1, p1-p1d/1
  Mux3/1 -> p1-p1d/2
  Inertia/1 -> Product/1
  Add1/1 -> Integrator/1, ddx_r1/1
  Product2/1 -> Add2/2
  Mux/1 -> k1(p1-p1d);2kapeta*q1/q1d/2
  Quaternion Division1/1 -> Scope2/1, Demux1/1
  Mux2/1 -> Quaternion Division1/1
  Mux4/1 -> Quaternion Division1/2
  k1(p1-p1d);2kapeta*q1/q1d/1 -> Add2/1
  Product/1 -> Add1/1
  Add2/1 -> Product/2
  ddx_d1/1 -> Scope4/1, Add1/2
  Demux3/2 -> Angular Velocity to Quaternion Orientation/1(omega_do)
  Demux3/1 -> Integrator1/1
  Integrator1/1 -> Mux5/1
  Integrator/1 -> Add/2, Scope9/1, Demux3/1, dx_r1/1
  Angular Velocity to Quaternion Orientation/1(q_do) -> Quaternion Normalize/1
  Quaternion Normalize/1 -> Mux5/2
  Mux5/1 -> Demux2/1, x_r1/1
  h_I1/1 -> Scope6/1, Add2/3

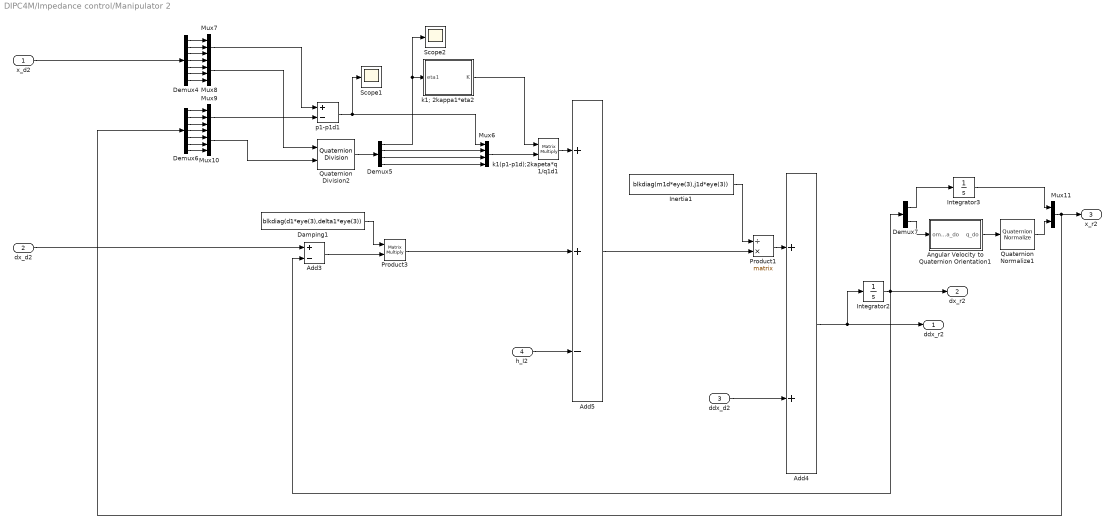
== system DIPC4M/Impedance control/Manipulator 2 ==
  x_d2 : Inport
  dx_d2 : Inport  Port=2
  ddx_d2 : Inport  Port=3
  h_I2 : Inport  Port=4
  Add3 : Sum  Inputs=+-
  Add4 : Sum
  Add5 : Sum  Inputs=++-
  Angular Velocity to Quaternion Orientation1 : Subsystem
  Damping1 : Constant  Value=blkdiag(d1*eye(3),delta1*eye(3))
  Demux4 : Demux  Outputs=7
  Demux5 : Demux
  Demux6 : Demux  Outputs=7
  Demux7 : Demux  Outputs=2
  Inertia1 : Constant  Value=blkdiag(m1d*eye(3),j1d*eye(3))
  Integrator2 : Integrator
  Integrator3 : Integrator  InitialCondition=r(4:6)
  Mux10 : Mux
  Mux11 : Mux  Inputs=2
  Mux6 : Mux
  Mux7 : Mux  Inputs=3
  Mux8 : Mux
  Mux9 : Mux  Inputs=3
  Product1 : Product  Inputs=/*  Multiplication=Matrix(*)
  Product3 : Product  Multiplication=Matrix(*)
  Quaternion Division2 : aerolibutil/Quaternion Division
  Quaternion Normalize1 : aerolibutil/Quaternion Normalize
  Scope1 : Scope
      settings: ShowLegends=on  TimeRange=200  YMin=-50  YMax=125  SaveName=ScopeData5
  Scope2 : Scope
      settings: ShowLegends=on  TimeRange=200  YMin=-50  YMax=125  SaveName=ScopeData13
  k1(p1-p1d);2kapeta*q1/q1d1 : Product  Multiplication=Matrix(*)
  k1; 2kappa1*eta2 : MATLAB Function  TreatAsAtomicUnit=on
  p1-p1d1 : Sum  Inputs=+-
  ddx_r2 : Outport
  dx_r2 : Outport  Port=2
  x_r2 : Outport  Port=3
  wires:
  Add3/1 -> Product3/2
  dx_d2/1 -> Add3/1
  Demux5/1 -> Scope2/1, k1; 2kappa1*eta2/1(eta1)
  k1; 2kappa1*eta2/1(K) -> k1(p1-p1d);2kapeta*q1/q1d1/1
  p1-p1d1/1 -> Scope1/1, Mux6/1
  Demux5/3 -> Mux6/3
  Demux5/2 -> Mux6/2
  Demux6/2 -> Mux9/2
  Demux5/4 -> Mux6/4
  x_d2/1 -> Demux4/1
  Demux4/3 -> Mux7/3
  Demux4/2 -> Mux7/2
  Damping1/1 -> Product3/1
  Demux4/1 -> Mux7/1
  Demux4/5 -> Mux8/2
  Demux4/4 -> Mux8/1
  Demux4/7 -> Mux8/4
  Demux4/6 -> Mux8/3
  Demux6/3 -> Mux9/3
  Demux6/1 -> Mux9/1
  Demux6/4 -> Mux10/1
  Demux6/6 -> Mux10/3
  Demux6/5 -> Mux10/2
  Demux6/7 -> Mux10/4
  Mux9/1 -> p1-p1d1/2
  Mux7/1 -> p1-p1d1/1
  Inertia1/1 -> Product1/1
  Add4/1 -> ddx_r2/1, Integrator2/1
  Product3/1 -> Add5/2
  Mux6/1 -> k1(p1-p1d);2kapeta*q1/q1d1/2
  Quaternion Division2/1 -> Demux5/1
  Mux8/1 -> Quaternion Division2/1
  Mux10/1 -> Quaternion Division2/2
  Product1/1 -> Add4/1
  k1(p1-p1d);2kapeta*q1/q1d1/1 -> Add5/1
  ddx_d2/1 -> Add4/2
  Add5/1 -> Product1/2
  Demux7/1 -> Integrator3/1
  Demux7/2 -> Angular Velocity to Quaternion Orientation1/1(omega_do)
  Integrator3/1 -> Mux11/1
  Integrator2/1 -> dx_r2/1, Add3/2, Demux7/1
  Angular Velocity to Quaternion Orientation1/1(q_do) -> Quaternion Normalize1/1
  Quaternion Normalize1/1 -> Mux11/2
  Mux11/1 -> x_r2/1, Demux6/1
  h_I2/1 -> Add5/3

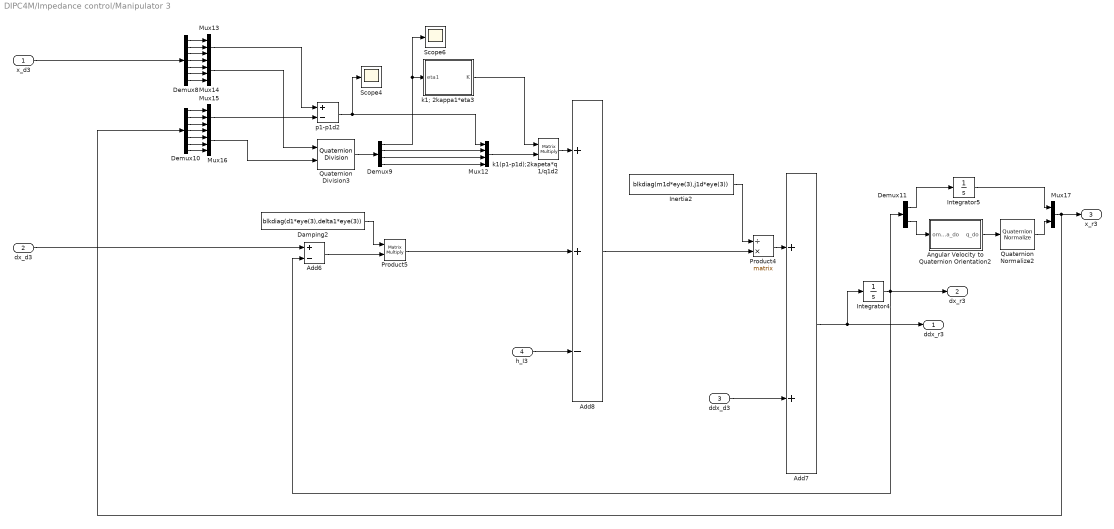
== system DIPC4M/Impedance control/Manipulator 3 ==
  x_d3 : Inport
  dx_d3 : Inport  Port=2
  ddx_d3 : Inport  Port=3
  h_I3 : Inport  Port=4
  Add6 : Sum  Inputs=+-
  Add7 : Sum
  Add8 : Sum  Inputs=++-
  Angular Velocity to Quaternion Orientation2 : Subsystem
  Damping2 : Constant  Value=blkdiag(d1*eye(3),delta1*eye(3))
  Demux10 : Demux  Outputs=7
  Demux11 : Demux  Outputs=2
  Demux8 : Demux  Outputs=7
  Demux9 : Demux
  Inertia2 : Constant  Value=blkdiag(m1d*eye(3),j1d*eye(3))
  Integrator4 : Integrator
  Integrator5 : Integrator  InitialCondition=r(7:9)
  Mux12 : Mux
  Mux13 : Mux  Inputs=3
  Mux14 : Mux
  Mux15 : Mux  Inputs=3
  Mux16 : Mux
  Mux17 : Mux  Inputs=2
  Product4 : Product  Inputs=/*  Multiplication=Matrix(*)
  Product5 : Product  Multiplication=Matrix(*)
  Quaternion Division3 : aerolibutil/Quaternion Division
  Quaternion Normalize2 : aerolibutil/Quaternion Normalize
  Scope4 : Scope
      settings: ShowLegends=on  TimeRange=200  YMin=-50  YMax=125  SaveName=ScopeData17
  Scope6 : Scope
      settings: ShowLegends=on  TimeRange=200  YMin=-50  YMax=125  SaveName=ScopeData19
  k1(p1-p1d);2kapeta*q1/q1d2 : Product  Multiplication=Matrix(*)
  k1; 2kappa1*eta3 : MATLAB Function  TreatAsAtomicUnit=on
  p1-p1d2 : Sum  Inputs=+-
  ddx_r3 : Outport
  dx_r3 : Outport  Port=2
  x_r3 : Outport  Port=3
  wires:
  Mux14/1 -> Quaternion Division3/1
  k1(p1-p1d);2kapeta*q1/q1d2/1 -> Add8/1
  Product4/1 -> Add7/1
  Mux16/1 -> Quaternion Division3/2
  Demux8/7 -> Mux14/4
  Demux10/1 -> Mux15/1
  Demux10/4 -> Mux16/1
  Angular Velocity to Quaternion Orientation2/1(q_do) -> Quaternion Normalize2/1
  Mux17/1 -> x_r3/1, Demux10/1
  k1; 2kappa1*eta3/1(K) -> k1(p1-p1d);2kapeta*q1/q1d2/1
  p1-p1d2/1 -> Scope4/1, Mux12/1
  Demux8/4 -> Mux14/1
  Demux10/2 -> Mux15/2
  Demux8/6 -> Mux14/3
  h_I3/1 -> Add8/3
  Demux10/3 -> Mux15/3
  Demux10/6 -> Mux16/3
  Demux10/5 -> Mux16/2
  Demux10/7 -> Mux16/4
  Add7/1 -> ddx_r3/1, Integrator4/1
  Mux13/1 -> p1-p1d2/1
  Mux15/1 -> p1-p1d2/2
  Quaternion Normalize2/1 -> Mux17/2
  Product5/1 -> Add8/2
  Mux12/1 -> k1(p1-p1d);2kapeta*q1/q1d2/2
  Quaternion Division3/1 -> Demux9/1
  dx_d3/1 -> Add6/1
  Add8/1 -> Product4/2
  Demux11/2 -> Angular Velocity to Quaternion Orientation2/1(omega_do)
  ddx_d3/1 -> Add7/2
  Demux9/1 -> Scope6/1, k1; 2kappa1*eta3/1(eta1)
  Damping2/1 -> Product5/1
  Demux9/2 -> Mux12/2
  Demux9/3 -> Mux12/3
  x_d3/1 -> Demux8/1
  Demux9/4 -> Mux12/4
  Demux8/2 -> Mux13/2
  Demux8/5 -> Mux14/2
  Demux8/1 -> Mux13/1
  Demux8/3 -> Mux13/3
  Inertia2/1 -> Product4/1
  Integrator5/1 -> Mux17/1
  Demux11/1 -> Integrator5/1
  Integrator4/1 -> dx_r3/1, Add6/2, Demux11/1
  Add6/1 -> Product5/2

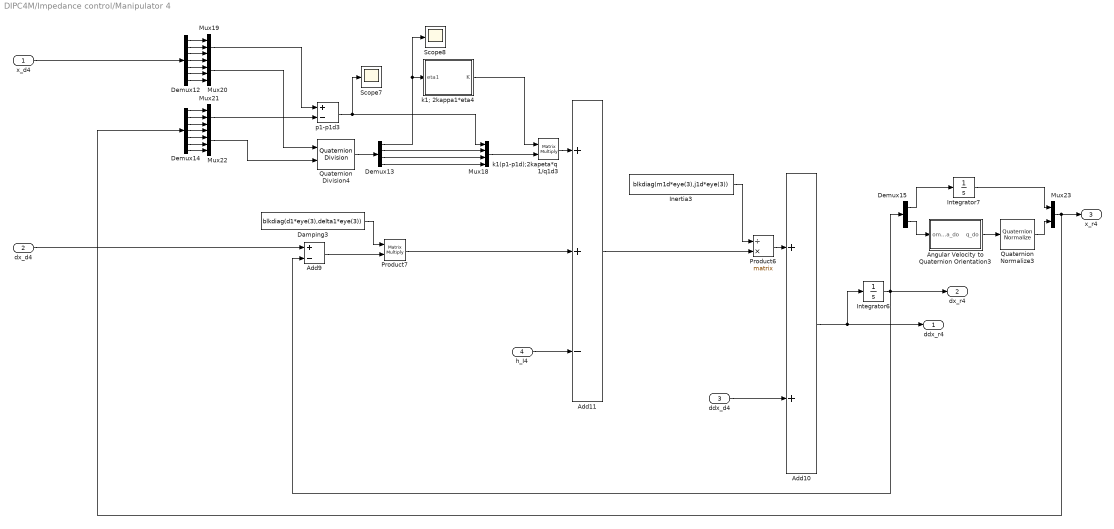
== system DIPC4M/Impedance control/Manipulator 4 ==
  x_d4 : Inport
  dx_d4 : Inport  Port=2
  ddx_d4 : Inport  Port=3
  h_I4 : Inport  Port=4
  Add10 : Sum
  Add11 : Sum  Inputs=++-
  Add9 : Sum  Inputs=+-
  Angular Velocity to Quaternion Orientation3 : Subsystem
  Damping3 : Constant  Value=blkdiag(d1*eye(3),delta1*eye(3))
  Demux12 : Demux  Outputs=7
  Demux13 : Demux
  Demux14 : Demux  Outputs=7
  Demux15 : Demux  Outputs=2
  Inertia3 : Constant  Value=blkdiag(m1d*eye(3),j1d*eye(3))
  Integrator6 : Integrator
  Integrator7 : Integrator  InitialCondition=r(10:12)
  Mux18 : Mux
  Mux19 : Mux  Inputs=3
  Mux20 : Mux
  Mux21 : Mux  Inputs=3
  Mux22 : Mux
  Mux23 : Mux  Inputs=2
  Product6 : Product  Inputs=/*  Multiplication=Matrix(*)
  Product7 : Product  Multiplication=Matrix(*)
  Quaternion Division4 : aerolibutil/Quaternion Division
  Quaternion Normalize3 : aerolibutil/Quaternion Normalize
  Scope7 : Scope
      settings: ShowLegends=on  TimeRange=200  YMin=-50  YMax=125  SaveName=ScopeData20
  Scope8 : Scope
      settings: ShowLegends=on  TimeRange=200  YMin=-50  YMax=125  SaveName=ScopeData22
  k1(p1-p1d);2kapeta*q1/q1d3 : Product  Multiplication=Matrix(*)
  k1; 2kappa1*eta4 : MATLAB Function  TreatAsAtomicUnit=on
  p1-p1d3 : Sum  Inputs=+-
  ddx_r4 : Outport
  dx_r4 : Outport  Port=2
  x_r4 : Outport  Port=3
  wires:
  dx_d4/1 -> Add9/1
  Demux13/1 -> Scope8/1, k1; 2kappa1*eta4/1(eta1)
  p1-p1d3/1 -> Scope7/1, Mux18/1
  Demux13/2 -> Mux18/2
  Demux13/3 -> Mux18/3
  Demux13/4 -> Mux18/4
  x_d4/1 -> Demux12/1
  Demux12/2 -> Mux19/2
  Demux12/1 -> Mux19/1
  Demux12/3 -> Mux19/3
  Demux12/4 -> Mux20/1
  Demux12/5 -> Mux20/2
  Demux12/6 -> Mux20/3
  Demux12/7 -> Mux20/4
  Demux14/2 -> Mux21/2
  Demux14/1 -> Mux21/1
  Demux14/3 -> Mux21/3
  Demux14/4 -> Mux22/1
  Demux14/5 -> Mux22/2
  Demux14/6 -> Mux22/3
  Demux14/7 -> Mux22/4
  Mux19/1 -> p1-p1d3/1
  Mux21/1 -> p1-p1d3/2
  Inertia3/1 -> Product6/1
  Add10/1 -> ddx_r4/1, Integrator6/1
  Product7/1 -> Add11/2
  Mux18/1 -> k1(p1-p1d);2kapeta*q1/q1d3/2
  Quaternion Division4/1 -> Demux13/1
  Mux20/1 -> Quaternion Division4/1
  Mux22/1 -> Quaternion Division4/2
  k1(p1-p1d);2kapeta*q1/q1d3/1 -> Add11/1
  Product6/1 -> Add10/1
  Add11/1 -> Product6/2
  ddx_d4/1 -> Add10/2
  Demux15/2 -> Angular Velocity to Quaternion Orientation3/1(omega_do)
  Demux15/1 -> Integrator7/1
  Integrator7/1 -> Mux23/1
  Integrator6/1 -> dx_r4/1, Add9/2, Demux15/1
  Angular Velocity to Quaternion Orientation3/1(q_do) -> Quaternion Normalize3/1
  Mux23/1 -> x_r4/1, Demux14/1
  Quaternion Normalize3/1 -> Mux23/2
  h_I4/1 -> Add11/3
  Add9/1 -> Product7/2
  Damping3/1 -> Product7/1
  k1; 2kappa1*eta4/1(K) -> k1(p1-p1d);2kapeta*q1/q1d3/1

== system DIPC4M/Manipulator motion/Angular Velocity to Quaternion ==
  omega_o : Inport
  Constant : Constant  Value=0
  Gain : Gain  Gain=0.5
  Integrator : Integrator  InitialCondition=[1; 0; 0; 0]
  Mux : Mux  Inputs=2
  Quaternion Multiplication : aerolibutil/Quaternion Multiplication
  Scope : Scope
      settings: ShowLegends=on  SaveName=ScopeData9
  q_o : Outport
  wires:
  omega_o/1 -> Gain/1
  Gain/1 -> Mux/2
  Constant/1 -> Mux/1
  Quaternion Multiplication/1 -> Integrator/1
  Integrator/1 -> Quaternion Multiplication/2, q_o/1, Scope/1
  Mux/1 -> Quaternion Multiplication/1

== system DIPC4M/Positional Control/Subsystem ==
  x_r : Inport
  x : Inport  Port=2
  Demux : Demux
  Demux1 : Demux
  Mux : Mux
  Subsystem : Subsystem
  Subsystem1 : Subsystem
  Subsystem2 : Subsystem
  Subsystem3 : Subsystem
  hk : Outport
  wires:
  x_r/1 -> Demux/1
  x/1 -> Demux1/1
  Demux/1 -> Subsystem/1(x_r1)
  Demux/2 -> Subsystem1/1(x_r2)
  Demux/3 -> Subsystem2/1(x_r3)
  Demux/4 -> Subsystem3/1(x_r4)
  Demux1/1 -> Subsystem/2(x1)
  Demux1/2 -> Subsystem1/2(x2)
  Demux1/3 -> Subsystem2/2(x3)
  Demux1/4 -> Subsystem3/2(x4)
  Subsystem/1(hk1) -> Mux/1
  Subsystem1/1(hk2) -> Mux/2
  Subsystem2/1(hk3) -> Mux/3
  Subsystem3/1(hk4) -> Mux/4
  Mux/1 -> hk/1

== system DIPC4M/Reference Trajectory/Angular Velocity to Quaternion Orientation ==
  omega_do : Inport
  Constant : Constant  Value=0
  Gain : Gain  Gain=0.5
  Integrator : Integrator  InitialCondition=[1; 0; 0; 0]
  Mux : Mux  Inputs=2
  Quaternion Multiplication : aerolibutil/Quaternion Multiplication
  Scope : Scope
      settings: ShowLegends=on  SaveName=ScopeData9
  q_do : Outport
  wires:
  omega_do/1 -> Gain/1
  Gain/1 -> Mux/2
  Constant/1 -> Mux/1
  Quaternion Multiplication/1 -> Integrator/1
  Integrator/1 -> Quaternion Multiplication/2, Scope/1, q_do/1
  Mux/1 -> Quaternion Multiplication/1

== system DIPC4M/Reference Trajectory/VIrtual Object Dynamics ==
  dx_do : Inport
  ddx_do : Inport  Port=2
  h_xo : Inport  Port=3
  Add : Sum  Inputs=+++
  Add1 : Sum  Inputs=-+
  Coriolis Force : MATLAB Function  TreatAsAtomicUnit=on
  Gravitation : Constant  Value=[-m0*g;zeros(3,1)]
  M_o*ddx_do : Product  Multiplication=Matrix(*)
  Object Inertia : Constant  Value=blkdiag(m0*eye(3),j0*eye(3));
  h_vo : Outport
  wires:
  Coriolis Force/1(hcoriolis) -> Add/2
  dx_do/1 -> Coriolis Force/1(dx_do)
  Gravitation/1 -> Add/1
  M_o*ddx_do/1 -> Add/3
  Object Inertia/1 -> M_o*ddx_do/1
  ddx_do/1 -> M_o*ddx_do/2
  Add/1 -> Add1/1
  h_xo/1 -> Add1/2
  Add1/1 -> h_vo/1

== system DIPC4M/Trajectory Generation/Angular Velocity to Quaternion Orientation ==
  omega_do : Inport
  Constant : Constant  Value=0
  Gain : Gain  Gain=0.5
  Integrator : Integrator  InitialCondition=[1; 0; 0; 0]
  Mux : Mux  Inputs=2
  Quaternion Multiplication : aerolibutil/Quaternion Multiplication
  Scope : Scope
      settings: ShowLegends=on  SaveName=ScopeData9
  q_do : Outport
  wires:
  omega_do/1 -> Gain/1
  Gain/1 -> Mux/2
  Constant/1 -> Mux/1
  Quaternion Multiplication/1 -> Integrator/1
  Integrator/1 -> Quaternion Multiplication/2, Scope/1, q_do/1
  Mux/1 -> Quaternion Multiplication/1

== system DIPC4M/Impedance control/Manipulator 1/Angular Velocity to Quaternion Orientation ==
  omega_do : Inport
  Constant : Constant  Value=0
  Gain : Gain  Gain=0.5
  Integrator : Integrator  InitialCondition=[1; 0; 0; 0]
  Mux : Mux  Inputs=2
  Quaternion Multiplication : aerolibutil/Quaternion Multiplication
  Scope : Scope
      settings: ShowLegends=on  SaveName=ScopeData9
  q_do : Outport
  wires:
  omega_do/1 -> Gain/1
  Gain/1 -> Mux/2
  Constant/1 -> Mux/1
  Quaternion Multiplication/1 -> Integrator/1
  Integrator/1 -> Quaternion Multiplication/2, Scope/1, q_do/1
  Mux/1 -> Quaternion Multiplication/1

== system DIPC4M/Impedance control/Manipulator 2/Angular Velocity to Quaternion Orientation1 ==
  omega_do : Inport
  Constant : Constant  Value=0
  Gain : Gain  Gain=0.5
  Integrator : Integrator  InitialCondition=[1; 0; 0; 0]
  Mux : Mux  Inputs=2
  Quaternion Multiplication : aerolibutil/Quaternion Multiplication
  Scope : Scope
      settings: ShowLegends=on  SaveName=ScopeData9
  q_do : Outport
  wires:
  omega_do/1 -> Gain/1
  Gain/1 -> Mux/2
  Constant/1 -> Mux/1
  Quaternion Multiplication/1 -> Integrator/1
  Integrator/1 -> Quaternion Multiplication/2, Scope/1, q_do/1
  Mux/1 -> Quaternion Multiplication/1

== system DIPC4M/Impedance control/Manipulator 3/Angular Velocity to Quaternion Orientation2 ==
  omega_do : Inport
  Constant : Constant  Value=0
  Gain : Gain  Gain=0.5
  Integrator : Integrator  InitialCondition=[1; 0; 0; 0]
  Mux : Mux  Inputs=2
  Quaternion Multiplication : aerolibutil/Quaternion Multiplication
  Scope : Scope
      settings: ShowLegends=on  SaveName=ScopeData9
  q_do : Outport
  wires:
  omega_do/1 -> Gain/1
  Gain/1 -> Mux/2
  Constant/1 -> Mux/1
  Quaternion Multiplication/1 -> Integrator/1
  Integrator/1 -> Quaternion Multiplication/2, Scope/1, q_do/1
  Mux/1 -> Quaternion Multiplication/1

== system DIPC4M/Impedance control/Manipulator 4/Angular Velocity to Quaternion Orientation3 ==
  omega_do : Inport
  Constant : Constant  Value=0
  Gain : Gain  Gain=0.5
  Integrator : Integrator  InitialCondition=[1; 0; 0; 0]
  Mux : Mux  Inputs=2
  Quaternion Multiplication : aerolibutil/Quaternion Multiplication
  Scope : Scope
      settings: ShowLegends=on  SaveName=ScopeData9
  q_do : Outport
  wires:
  omega_do/1 -> Gain/1
  Gain/1 -> Mux/2
  Constant/1 -> Mux/1
  Quaternion Multiplication/1 -> Integrator/1
  Integrator/1 -> Quaternion Multiplication/2, Scope/1, q_do/1
  Mux/1 -> Quaternion Multiplication/1

== system DIPC4M/Positional Control/Subsystem/Subsystem ==
  x_r1 : Inport
  x1 : Inport  Port=2
  Add1 : Sum  Inputs=+-
  Demux1 : Demux
  Demux2 : Demux  Outputs=7
  Demux3 : Demux  Outputs=7
  Mux : Mux
  Mux1 : Mux  Inputs=3
  Mux2 : Mux
  Mux3 : Mux  Inputs=3
  Mux4 : Mux
  Prod : Product  Multiplication=Matrix(*)
  Quaternion Division1 : aerolibutil/Quaternion Division
  k1; 2kappa1*eta1 : MATLAB Function  TreatAsAtomicUnit=on
  hk1 : Outport
  wires:
  k1; 2kappa1*eta1/1(K) -> Prod/1
  Demux1/1 -> k1; 2kappa1*eta1/1(eta1)
  Mux/1 -> Prod/2
  Quaternion Division1/1 -> Demux1/1
  Prod/1 -> hk1/1
  Demux1/4 -> Mux/4
  Demux1/3 -> Mux/3
  Demux1/2 -> Mux/2
  Demux2/1 -> Mux1/1
  Demux2/2 -> Mux1/2
  Demux2/3 -> Mux1/3
  Demux2/4 -> Mux2/1
  Demux2/5 -> Mux2/2
  Demux2/6 -> Mux2/3
  Demux2/7 -> Mux2/4
  x_r1/1 -> Demux2/1
  Demux3/1 -> Mux3/1
  Demux3/2 -> Mux3/2
  Demux3/3 -> Mux3/3
  Demux3/4 -> Mux4/1
  Demux3/5 -> Mux4/2
  Demux3/6 -> Mux4/3
  Demux3/7 -> Mux4/4
  x1/1 -> Demux3/1
  Mux1/1 -> Add1/1
  Mux3/1 -> Add1/2
  Mux2/1 -> Quaternion Division1/1
  Mux4/1 -> Quaternion Division1/2
  Add1/1 -> Mux/1

== system DIPC4M/Positional Control/Subsystem/Subsystem1 ==
  x_r2 : Inport
  x2 : Inport  Port=2
  Add2 : Sum  Inputs=+-
  Demux4 : Demux
  Demux5 : Demux  Outputs=7
  Demux6 : Demux  Outputs=7
  Mux5 : Mux
  Mux6 : Mux  Inputs=3
  Mux7 : Mux
  Mux8 : Mux  Inputs=3
  Mux9 : Mux
  Prod1 : Product  Multiplication=Matrix(*)
  Quaternion Division2 : aerolibutil/Quaternion Division
  k1; 2kappa1*eta2 : MATLAB Function  TreatAsAtomicUnit=on
  hk2 : Outport
  wires:
  Demux5/6 -> Mux7/3
  Demux6/1 -> Mux8/1
  x_r2/1 -> Demux5/1
  Demux6/3 -> Mux8/3
  Demux6/2 -> Mux8/2
  Demux6/5 -> Mux9/2
  Demux6/4 -> Mux9/1
  Demux6/7 -> Mux9/4
  Demux6/6 -> Mux9/3
  Mux6/1 -> Add2/1
  x2/1 -> Demux6/1
  Mux7/1 -> Quaternion Division2/1
  Mux8/1 -> Add2/2
  Add2/1 -> Mux5/1
  Mux9/1 -> Quaternion Division2/2
  k1; 2kappa1*eta2/1(K) -> Prod1/1
  Demux4/1 -> k1; 2kappa1*eta2/1(eta2)
  Mux5/1 -> Prod1/2
  Quaternion Division2/1 -> Demux4/1
  Prod1/1 -> hk2/1
  Demux4/4 -> Mux5/4
  Demux4/3 -> Mux5/3
  Demux4/2 -> Mux5/2
  Demux5/1 -> Mux6/1
  Demux5/2 -> Mux6/2
  Demux5/3 -> Mux6/3
  Demux5/4 -> Mux7/1
  Demux5/7 -> Mux7/4
  Demux5/5 -> Mux7/2

== system DIPC4M/Positional Control/Subsystem/Subsystem2 ==
  x_r3 : Inport
  x3 : Inport  Port=2
  Add3 : Sum  Inputs=+-
  Demux7 : Demux
  Demux8 : Demux  Outputs=7
  Demux9 : Demux  Outputs=7
  Mux10 : Mux
  Mux11 : Mux  Inputs=3
  Mux12 : Mux
  Mux13 : Mux  Inputs=3
  Mux14 : Mux
  Prod2 : Product  Multiplication=Matrix(*)
  Quaternion Division3 : aerolibutil/Quaternion Division
  k1; 2kappa1*eta3 : MATLAB Function  TreatAsAtomicUnit=on
  hk3 : Outport
  wires:
  Demux7/1 -> k1; 2kappa1*eta3/1(eta3)
  Prod2/1 -> hk3/1
  Demux8/1 -> Mux11/1
  Demux7/3 -> Mux10/3
  Demux7/2 -> Mux10/2
  Quaternion Division3/1 -> Demux7/1
  Mux10/1 -> Prod2/2
  Demux7/4 -> Mux10/4
  Demux8/7 -> Mux12/4
  Demux9/2 -> Mux13/2
  Demux9/1 -> Mux13/1
  Demux8/2 -> Mux11/2
  Demux8/3 -> Mux11/3
  Demux8/4 -> Mux12/1
  x_r3/1 -> Demux8/1
  Demux8/5 -> Mux12/2
  Demux8/6 -> Mux12/3
  Demux9/5 -> Mux14/2
  Demux9/7 -> Mux14/4
  Mux11/1 -> Add3/1
  k1; 2kappa1*eta3/1(K) -> Prod2/1
  x3/1 -> Demux9/1
  Add3/1 -> Mux10/1
  Mux13/1 -> Add3/2
  Mux12/1 -> Quaternion Division3/1
  Mux14/1 -> Quaternion Division3/2
  Demux9/4 -> Mux14/1
  Demux9/3 -> Mux13/3
  Demux9/6 -> Mux14/3

== system DIPC4M/Positional Control/Subsystem/Subsystem3 ==
  x_r4 : Inport
  x4 : Inport  Port=2
  Add4 : Sum  Inputs=+-
  Demux10 : Demux
  Demux11 : Demux  Outputs=7
  Demux12 : Demux  Outputs=7
  Mux15 : Mux
  Mux16 : Mux  Inputs=3
  Mux17 : Mux
  Mux18 : Mux  Inputs=3
  Mux19 : Mux
  Prod3 : Product  Multiplication=Matrix(*)
  Quaternion Division4 : aerolibutil/Quaternion Division
  k1; 2kappa1*eta4 : MATLAB Function  TreatAsAtomicUnit=on
  hk4 : Outport
  wires:
  k1; 2kappa1*eta4/1(K) -> Prod3/1
  Demux10/1 -> k1; 2kappa1*eta4/1(eta4)
  Mux15/1 -> Prod3/2
  Quaternion Division4/1 -> Demux10/1
  Prod3/1 -> hk4/1
  Demux10/4 -> Mux15/4
  Demux10/3 -> Mux15/3
  Demux10/2 -> Mux15/2
  Demux11/1 -> Mux16/1
  Demux11/2 -> Mux16/2
  Demux11/3 -> Mux16/3
  Demux11/4 -> Mux17/1
  Demux11/5 -> Mux17/2
  Demux11/6 -> Mux17/3
  Demux11/7 -> Mux17/4
  x_r4/1 -> Demux11/1
  Demux12/1 -> Mux18/1
  Demux12/2 -> Mux18/2
  Demux12/3 -> Mux18/3
  Demux12/4 -> Mux19/1
  Demux12/5 -> Mux19/2
  Demux12/6 -> Mux19/3
  Demux12/7 -> Mux19/4
  x4/1 -> Demux12/1
  Mux16/1 -> Add4/1
  Mux18/1 -> Add4/2
  Mux17/1 -> Quaternion Division4/1
  Mux19/1 -> Quaternion Division4/2
  Add4/1 -> Mux15/1

== matlab function DIPC4M/Reference Trajectory/MATLAB Function1 ==
  data: eta_o input; K output; K_o parameter; kappa_o parameter
function K = stiffness(eta_o,K_o,kappa_o)
K = blkdiag(K_o*eye(3),2*eta_o*kappa_o*eye(3));

== matlab function DIPC4M/Reference Trajectory/Grasp Matrix ==
  data: r parameter; G output; x input size=28
function G = GraspMatrix(r,x)
%x_o = [eye(3) zeros(3,4) eye(3) zeros(3,4) eye(3) zeros(3,4) eye(3) zeros(3,4)] * x;
G = [eye(3) zeros(3) eye(3) zeros(3) eye(3) zeros(3) eye(3) zeros(3);
    skew_sm(quatrot(x(4:7),r(1:3))) eye(3) skew_sm(quatrot(x(4:7),r(4:6))) eye(3) skew_sm(quatrot(x(4:7),r(7:9))) eye(3) skew_sm(quatrot(x(4:7),r(10:12))) eye(3)];

== matlab function DIPC4M/Reference Trajectory/Coriolis Force ==
  data: dx_do input; hcoriolis output; j0 parameter; m0 parameter
function hcoriolis = CoriolisForce(dx_do,j0,m0)
hcoriolis = [m0*skew_sm(dx_do(4:6))*dx_do(1:3);
        j0*skew_sm(dx_do(4:6))*dx_do(4:6)];
